simulink model "lab1_model_challenge_robustSS_windup"  (R2024b)
settings: Solver=ode45  StartTime=0.0  StopTime=sIn.simulation_time
undefined symbols (not defined in the file or in its folder): degs2rpm, feedback, filt, rpm2rads, sens
libraries: simulink x1
settings Model: Creator=bmm1  LastModifiedBy=pries
settings DataIOCC: ReturnWorkspaceOutputs=off
settings RTWCC: GPUComputeCapability=3.5

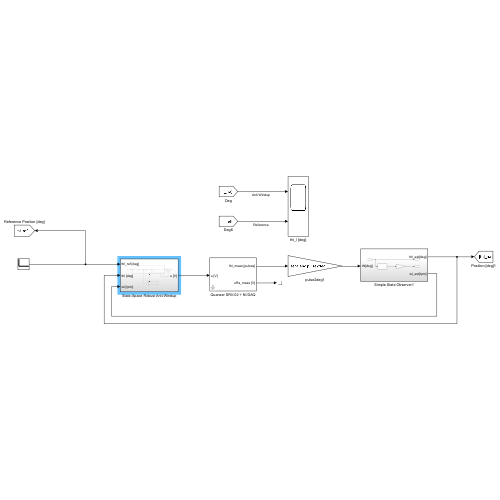
[thumbnail: Simulink's stored preview of the top-level diagram]
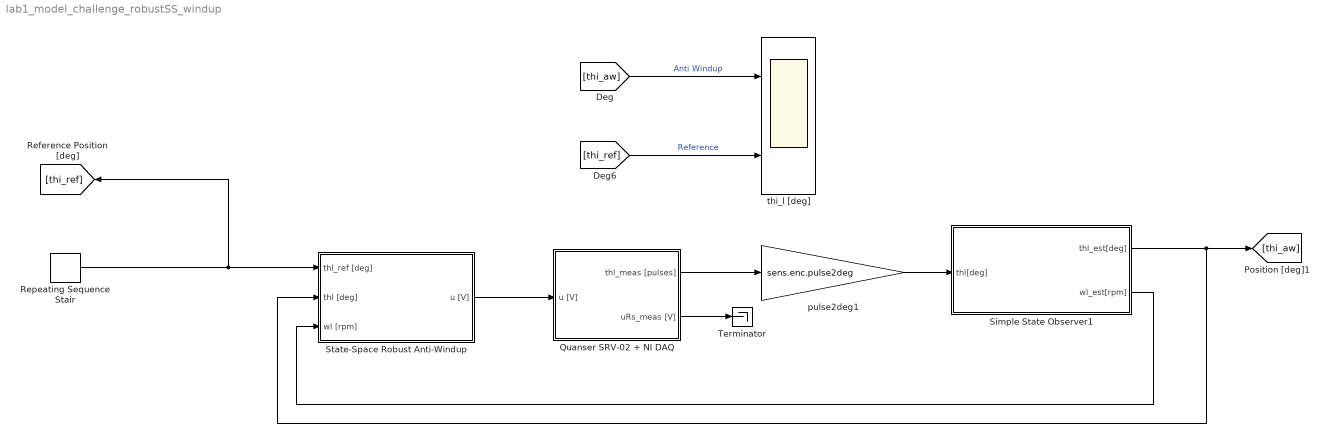
== system lab1_model_challenge_robustSS_windup ==
  Quanser SRV-02 + NI DAQ : Subsystem  mask(Quanser SRV-02 (with inertial load) + NI DAQ){Ts=0.001, fricType=Coulomb + viscous}
      mask prompts: Ts "NI DAQ Sample Time:"; fricType "Friction model"
      mask help: Quanser SRV-02 (with inertial load) + NI DAQ model.
      mask init:
      | %%  Sensors data
      | 
      | %   shunt resistor
      | sens.curr.Rs = 0.5;                         %   resistance [Ohm]   
      | sens.curr.uRs_std = 0.01;                   %   voltage noise standard dev [V]                           
      | sens.curr.uRs_var = sens.curr.uRs_std^2;	%   voltage noise variance [V^2]
      | 
      | %   Hewlett-Packard HEDS-5540#A06 optical encoder
      | sens.enc.ppr = 500*4;                       %   pulses per rotation
      | sens.enc.pulse2deg = 360/sens.enc.ppr;      %   [pulses] -> [deg]
      | sens.enc.pulse2rad = 2*pi/sens.enc.ppr;     %   [pulses] -> [rad]
      | sens.enc.deg2pulse = sens.enc.ppr/360;      %   [deg] -> [pulses]
      | sens.enc.rad2pulse = sens.enc.ppr/2/pi;     %   [rad] -> [pulses]
      | 
      | 
      | %%  Data acquisition board (daq) data
      | 
      | %   NI PCI-6221 DAC data
      | daq.dac.bits = 16;                                  %   resolution (bits)
      | daq.dac.fs   = 10;                                  %   full scale 
      | daq.dac.q    = 2*daq.dac.fs/(2^daq.dac.bits-1);     %	quantization
      | 
      | %   NI PCI-6221 ADC data
      | daq.adc.bits = 16;                                  %   resolution (bits)
      | daq.adc.fs   = 10;                                  %   full scale (as set in SLDRT Analog Input block)
      | daq.adc.q    = 2*daq.adc.fs/(2^daq.adc.bits-1);     %   quantization
      mask Help:
      | Riccardo Antonello (antonello@dei.unipd.it)
      | 
      | April 24, 2020
      | 
      | Dept. of Information Engineering, University of Padova
      mask TypeOptions fricType: Coulomb + viscous | Karnopp
  Repeating Sequence Stair : simulink/Sources/Repeating Sequence Stair  OutValues=sIn.position  tsamp=sIn.sample_time  OutMin=[]  OutMax=[]  OutDataTypeStr=double  OutputDataTypeScalingMode=double  OutDataType=fixdt(0,8)  ConRadixGroup=Best Precision: Vector-wise  OutScaling=2^-12
  Simple State Observer1 : Subsystem
  State-Space Robust Anti-Windup : Subsystem
  Terminator : Terminator
  pulse2deg1 : Gain  Gain=sens.enc.pulse2deg
  thi_l [deg] : Scope  NumInputPorts=2
  wires:
  Repeating Sequence Stair/1 -> [thi_ref], State-Space Robust Anti-Windup/1(thl_ref [deg])
  State-Space Robust Anti-Windup/1(u [V]) -> Quanser SRV-02 + NI DAQ/1(u [V])
  Quanser SRV-02 + NI DAQ/1(thl_meas [pulses]) -> pulse2deg1/1
  Simple State Observer1/1(thl_est[deg]) -> State-Space Robust Anti-Windup/2(thl [deg]), [thi_aw]
  Simple State Observer1/2(wl_est[rpm]) -> State-Space Robust Anti-Windup/3(wl [rpm])
  [thi_aw] -> thi_l [deg]/1  "Anti Windup"
  [thi_ref] -> thi_l [deg]/2  "Reference"
  pulse2deg1/1 -> Simple State Observer1/1(thl[deg])
  Quanser SRV-02 + NI DAQ/2(uRs_meas [V]) -> Terminator/1

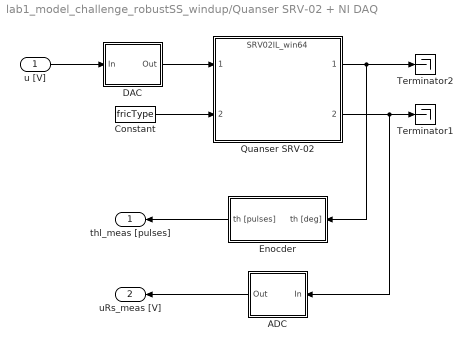
== system lab1_model_challenge_robustSS_windup/Quanser SRV-02 + NI DAQ ==
  u [V] : Inport
  ADC : Subsystem
  Constant : Constant  Value=fricType
  DAC : Subsystem
  Enocder : Subsystem
  Quanser SRV-02 : ModelReference  ModelNameDialog=SRV02IL_win64.slxp  ModelReferenceVersion=1.44  CopyOfModelProtected=on
  Terminator1 : Terminator
  Terminator2 : Terminator
  thl_meas [pulses] : Outport
  uRs_meas [V] : Outport  Port=2
  wires:
  Enocder/1(th [pulses]) -> thl_meas [pulses]/1
  ADC/1(Out) -> uRs_meas [V]/1
  DAC/1(Out) -> Quanser SRV-02/1
  Quanser SRV-02/2 -> ADC/1(In), Terminator1/1
  u [V]/1 -> DAC/1(In)
  Quanser SRV-02/1 -> Enocder/1(th [deg]), Terminator2/1
  Constant/1 -> Quanser SRV-02/2

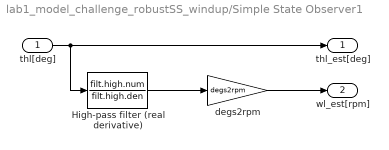
== system lab1_model_challenge_robustSS_windup/Simple State Observer1 ==
  thl[deg] : Inport
  High-pass filter (real derivative) : TransferFcn  Numerator=filt.high.num  Denominator=filt.high.den
  degs2rpm : Gain  Gain=degs2rpm
  thl_est[deg] : Outport
  wl_est[rpm] : Outport  Port=2
  wires:
  thl[deg]/1 -> High-pass filter (real derivative)/1, thl_est[deg]/1
  High-pass filter (real derivative)/1 -> degs2rpm/1
  degs2rpm/1 -> wl_est[rpm]/1

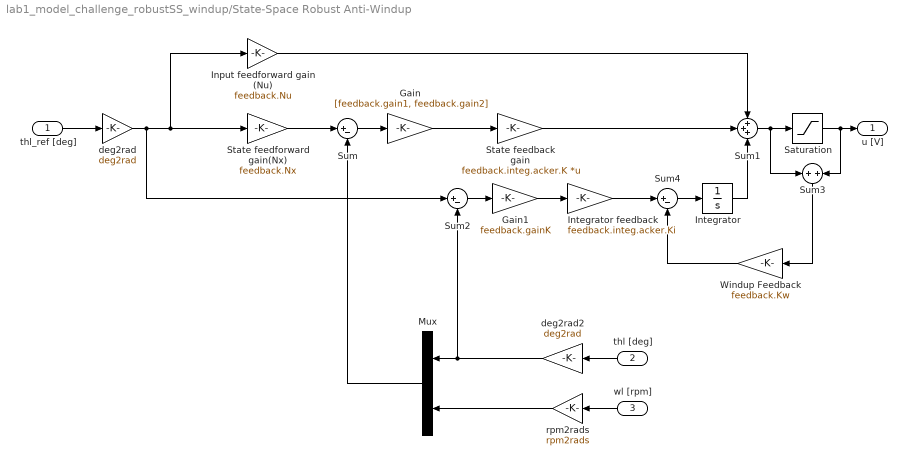
== system lab1_model_challenge_robustSS_windup/State-Space Robust Anti-Windup ==
  thl_ref [deg] : Inport
  thl [deg] : Inport  Port=2
  wl [rpm] : Inport  Port=3
  Gain : Gain  Gain=[feedback.gain1, feedback.gain2]
  Gain1 : Gain  Gain=feedback.gainK
  Input feedforward gain (Nu) : Gain  Gain=feedback.Nu
  Integrator : Integrator
  Integrator feedback : Gain  Gain=feedback.integ.acker.Ki
  Mux : Mux  Inputs=2
  Saturation : Saturate  UpperLimit=10  LowerLimit=-10
  State feedback gain : Gain  Gain=feedback.integ.acker.K  Multiplication=Matrix(K*u)
  State feedforward gain(Nx) : Gain  Gain=feedback.Nx
  Sum : Sum  Inputs=|+-
  Sum1 : Sum  Inputs=+++
  Sum2 : Sum  Inputs=|+-
  Sum3 : Sum  Inputs=+|+
  Sum4 : Sum  Inputs=|+-
  Windup Feedback : Gain  Gain=feedback.Kw
  deg2rad : Gain  Gain=deg2rad
  deg2rad2 : Gain  Gain=deg2rad
  rpm2rads : Gain  Gain=rpm2rads
  u [V] : Outport
  wires:
  thl_ref [deg]/1 -> deg2rad/1
  deg2rad/1 -> Sum2/1, Input feedforward gain (Nu)/1, State feedforward gain(Nx)/1
  State feedforward gain(Nx)/1 -> Sum/1
  Sum/1 -> Gain/1
  State feedback gain/1 -> Sum1/2
  Input feedforward gain (Nu)/1 -> Sum1/1
  Sum1/1 -> Sum3/1, Saturation/1
  Saturation/1 -> Sum3/2, u [V]/1
  thl [deg]/1 -> deg2rad2/1
  wl [rpm]/1 -> rpm2rads/1
  deg2rad2/1 -> Mux/1, Sum2/2
  rpm2rads/1 -> Mux/2
  Mux/1 -> Sum/2
  Sum2/1 -> Gain1/1
  Integrator/1 -> Sum1/3
  Sum3/1 -> Windup Feedback/1
  Integrator feedback/1 -> Sum4/1
  Sum4/1 -> Integrator/1
  Windup Feedback/1 -> Sum4/2
  Gain/1 -> State feedback gain/1
  Gain1/1 -> Integrator feedback/1

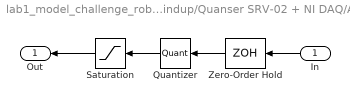
== system lab1_model_challenge_robustSS_windup/Quanser SRV-02 + NI DAQ/ADC ==
  In : Inport
  Quantizer : Quantizer  QuantizationInterval=daq.adc.q
  Saturation : Saturate  UpperLimit=daq.adc.fs  LowerLimit=-daq.adc.fs
  Zero-Order Hold : ZeroOrderHold  SampleTime=Ts
  Out : Outport
  wires:
  Saturation/1 -> Out/1
  In/1 -> Zero-Order Hold/1
  Quantizer/1 -> Saturation/1
  Zero-Order Hold/1 -> Quantizer/1

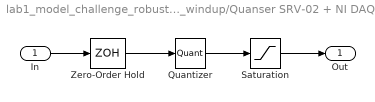
== system lab1_model_challenge_robustSS_windup/Quanser SRV-02 + NI DAQ/DAC ==
  In : Inport
  Quantizer : Quantizer  QuantizationInterval=daq.dac.q
  Saturation : Saturate  UpperLimit=daq.dac.fs  LowerLimit=-daq.dac.fs
  Zero-Order Hold : ZeroOrderHold  SampleTime=Ts
  Out : Outport
  wires:
  Quantizer/1 -> Saturation/1
  In/1 -> Zero-Order Hold/1
  Zero-Order Hold/1 -> Quantizer/1
  Saturation/1 -> Out/1

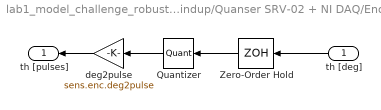
== system lab1_model_challenge_robustSS_windup/Quanser SRV-02 + NI DAQ/Enocder ==
  th [deg] : Inport
  Quantizer : Quantizer  QuantizationInterval=sens.enc.pulse2deg
  Zero-Order Hold : ZeroOrderHold  SampleTime=Ts
  deg2pulse : Gain  Gain=sens.enc.deg2pulse
  th [pulses] : Outport
  wires:
  Quantizer/1 -> deg2pulse/1
  th [deg]/1 -> Zero-Order Hold/1
  Zero-Order Hold/1 -> Quantizer/1
  deg2pulse/1 -> th [pulses]/1
